simulink model "DLCReferenceApplication"  (R2023a)
settings: Solver=ode23tb  StartTime=0.0  StopTime=25  FixedStep=.001  RelTol=2e-1  EnableMultiTasking=on
StartFcn:
  | %tic
StopFcn:
  | %toc
model workspace (MAT data in the model file):
  DLCXref = [0 6.1 6.2 18 33 33.5 45 50 60]
  DLCXrefStanley = [0 1.2 2.4 3.6 4.8 6 7.2 8.4 9.44987166868 10.0991210544 10.1 10.1008789456 10.7501283313 11.8 15.24 18.68 22.12 25.56 29 31.0586706708 32.3317697631 32.5 33.2655829029 35.0745965915 36 38.7142857143 41.4285714286 44.1428571429 46.8571428571 49.5714285714 52.2857142857 55 55.7142857143 56.4285714286 57.1428571429 57.8571428571 58.5714285714 59.2857142857]
  DLCYref = [0 0 -5 -3.875 -3.5 1 0 0 0]
  DLCYrefStanley = [0.1375 0.1375 0.1375 0.1375 0.1375 0.1375 0.1375 0.1375 -0.203439148031 -1.09615705337 -2.2 -3.30384294663 -4.19656085197 -4.5375 -4.5375 -4.5375 -4.5375 -4.5375 -4.5375 -3.86895979121 -2.11844853934 -1.2 0.824587306188 2.01309074174 2.1375 1.85178571429 1.56607142857 1.28035714286 0.994642857143 0.708928571429 0.423214285714 0.1375 0.1375 0.1375 0.1375 0.1375 0.1375 0.1375]
  Downshift_Speeds = [9.5625  23.0625  36.5625  47.8125  59.0625  68.90625  78.75; 12.9375  26.4375  39.9375  51.1875  62.4375  72.84375  83.25; 16.3125  29.8125  43.3125  54.5625  65.8125  76.78125  87.75; 19.6875  33.1875  46.6875  57.9375  69.1875  80.71875  92.25]
  EngRevLim = 7000
  Pedal_Positions = [0.1 0.4 0.5 0.9]
  Upshift_Speeds = [12.9375  26.4375  39.9375  51.1875  62.4375  72.84375  83.25; 16.3125  29.8125  43.3125  54.5625  65.8125  76.78125  87.75; 19.6875  33.1875  46.6875  57.9375  69.1875  80.71875  92.25; 33  52.5  77.25  100.5  138.75  161.875  185]
  VEH.Mass = 1181
  VEH.StaticNormalFrontLoad.FR = 264.666666667
  VEH.StaticNormalFrontLoad.FL = 264.666666667
  VEH.StaticNormalRearLoad.RR = 322
  VEH.StaticNormalRearLoad.RL = 322
  VEH.WheelBase = 3.075
  VEH.FrontAxlePositionfromCG = 1.515
  VEH.RearAxlePositionfromCG = 1.504
  VEH.HeightCG = 0.134
  VEH.FrontalArea = 2.11
  VEH.DragCoefficient = 0.33
  VEH.NumberOfWheelsPerAxle = 2
  VEH.PitchMomentInertia = 1922.66666667
  VEH.RollMomentInertia = 432.333333333
  VEH.YawMomentInertia = 2066
  VEH.SteeringRatio = 18
  VEH.TrackWidth = 1.922
  VEH.SprungMass = 1096.72266667
  VEH.InitialLongPosition = 0
  VEH.InitialLatPosition = 5.7
  VEH.InitialVertPosition = 0
  VEH.InitialRollAngle = 0
  VEH.InitialPitchAngle = 0
  VEH.InitialYawAngle = 0
  VEH.InitialLongVel = 0
  VEH.InitialLatVel = 0
  VEH.InitialVertVel = 0
  VEH.InitialRollRate = 0
  VEH.InitialPitchRate = 0
  VEH.InitialYawRate = 0
  VEH.UnsprungMassRearAxle = 160
  VEH.UnsprungMassFrontAxle = 100
  rayDirections = [0  0  -1; 0  0  -1; 0  0  -1; 0  0  -1; 0  0  -1; 0  0  -1; 0  0  -1; 0  0  -1; 0  0  -1; 0  0  -1; 0  0  -1; 0  0  -1; 0  0  -1; 0  0  -1; 0  0  -1; 0  0  -1; 0  0  -1; 0  0  -1; 0  0  -1; 0  0  -1; 0  0  -1; 0  0  -1; 0  0  -1; 0  0  -1; 0  0  -1; 0  0  -1; 0  0  -1; 0  0  -1; 0  0  -1; 0  0  -1; 0  0  -1; 0  0  -1; 0  0  -1; 0  0  -1; 0  0  -1; 0  0  -1; 0  0  -1; 0  0  -1; 0  0  -1; 0  0  -1; 0  0  -1; 0  0  -1; 0  0  -1; 0  0  -1; 0  0  -1; 0  0  -1; 0  0  -1; 0  0  -1; 0  0  -1; 0  0  -1; 0  0  -1; 0  0  -1; 0  0  -1; 0  0  -1; 0  0  -1; 0  0  -1; 0  0  -1; 0  0  -1; 0  0  -1; 0  0  -1; 0  0  -1; 0  0  -1; 0  0  -1; 0  0  -1; 0  0  -1; 0  0  -1; 0  0  -1; 0  0  -1; 0  0  -1; 0  0  -1; 0  0  -1; 0  0  -1; 0  0  -1; 0  0  -1; 0  0  -1; 0  0  -1; 0  0  -1; 0  0  -1; 0  0  -1; 0  0  -1; 0  0  -1; 0  0  -1; 0  0  -1; 0  0  -1; 0  0  -1; 0  0  -1; 0  0  -1; 0  0  -1; 0  0  -1; 0  0  -1; 0  0  -1; 0  0  -1; 0  0  -1; 0  0  -1; 0  0  -1; 0  0  -1; 0  0  -1; 0  0  -1; 0  0  -1; 0  0  -1; 0  0  -1; 0  0  -1; 0  0  -1; 0  0  -1; 0  0  -1; 0  0  -1; 0  0  -1; 0  0  -1; 0  0  -1; 0  0  -1; 0  0  -1; 0  0  -1; 0  0  -1; 0  0  -1; 0  0  -1; 0  0  -1; 0  0  -1; 0  0  -1; 0  0  -1; 0  0  -1; 0  0  -1]
  rayLengths = [20; 20; 20; 20; 20; 20; 20; 20; 20; 20; 20; 20; 20; 20; 20; 20; 20; 20; 20; 20; 20; 20; 20; 20; 20; 20; 20; 20; 20; 20; 20; 20; 20; 20; 20; 20; 20; 20; 20; 20; 20; 20; 20; 20; 20; 20; 20; 20; 20; 20; 20; 20; 20; 20; 20; 20; 20; 20; 20; 20; 20; 20; 20; 20; 20; 20; 20; 20; 20; 20; 20; 20; 20; 20; 20; 20; 20; 20; 20; 20; 20; 20; 20; 20; 20; 20; 20; 20; 20; 20; 20; 20; 20; 20; 20; 20; 20; 20; 20; 20; 20; 20; 20; 20; 20; 20; 20; 20; 20; 20; 20; 20; 20; 20; 20; 20; 20; 20; 20; 20; 20]
  rayOrigins = [0.5  -0.5  0; 0.4  -0.5  0; 0.3  -0.5  0; 0.2  -0.5  0; 0.1  -0.5  0; 0  -0.5  0; -0.1  -0.5  0; -0.2  -0.5  0; -0.3  -0.5  0; -0.4  -0.5  0; -0.5  -0.5  0; 0.5  -0.4  0; 0.4  -0.4  0; 0.3  -0.4  0; 0.2  -0.4  0; 0.1  -0.4  0; 0  -0.4  0; -0.1  -0.4  0; -0.2  -0.4  0; -0.3  -0.4  0; -0.4  -0.4  0; -0.5  -0.4  0; 0.5  -0.3  0; 0.4  -0.3  0; 0.3  -0.3  0; 0.2  -0.3  0; 0.1  -0.3  0; 0  -0.3  0; -0.1  -0.3  0; -0.2  -0.3  0; -0.3  -0.3  0; -0.4  -0.3  0; -0.5  -0.3  0; 0.5  -0.2  0; 0.4  -0.2  0; 0.3  -0.2  0; 0.2  -0.2  0; 0.1  -0.2  0; 0  -0.2  0; -0.1  -0.2  0; -0.2  -0.2  0; -0.3  -0.2  0; -0.4  -0.2  0; -0.5  -0.2  0; 0.5  -0.1  0; 0.4  -0.1  0; 0.3  -0.1  0; 0.2  -0.1  0; 0.1  -0.1  0; 0  -0.1  0; -0.1  -0.1  0; -0.2  -0.1  0; -0.3  -0.1  0; -0.4  -0.1  0; -0.5  -0.1  0; 0.5  0  0; 0.4  0  0; 0.3  0  0; 0.2  0  0; 0.1  0  0; 0  0  0; -0.1  0  0; -0.2  0  0; -0.3  0  0; -0.4  0  0; -0.5  0  0; 0.5  0.1  0; 0.4  0.1  0; 0.3  0.1  0; 0.2  0.1  0; 0.1  0.1  0; 0  0.1  0; -0.1  0.1  0; -0.2  0.1  0; -0.3  0.1  0; -0.4  0.1  0; -0.5  0.1  0; 0.5  0.2  0; 0.4  0.2  0; 0.3  0.2  0; 0.2  0.2  0; 0.1  0.2  0; 0  0.2  0; -0.1  0.2  0; -0.2  0.2  0; -0.3  0.2  0; -0.4  0.2  0; -0.5  0.2  0; 0.5  0.3  0; 0.4  0.3  0; 0.3  0.3  0; 0.2  0.3  0; 0.1  0.3  0; 0  0.3  0; -0.1  0.3  0; -0.2  0.3  0; -0.3  0.3  0; -0.4  0.3  0; -0.5  0.3  0; 0.5  0.4  0; 0.4  0.4  0; 0.3  0.4  0; 0.2  0.4  0; 0.1  0.4  0; 0  0.4  0; -0.1  0.4  0; -0.2  0.4  0; -0.3  0.4  0; -0.4  0.4  0; -0.5  0.4  0; 0.5  0.5  0; 0.4  0.5  0; 0.3  0.5  0; 0.2  0.5  0; 0.1  0.5  0; 0  0.5  0; -0.1  0.5  0; -0.2  0.5  0; -0.3  0.5  0; -0.4  0.5  0; -0.5  0.5  0]
undefined symbols (not defined in the file or in its folder): DiscIntNeverNeededParam
libraries: simulink x14, autolibutils x7, vehdynlibdriver x2, vehdynlibviscommon x2, sim3dgroundtruthsensorlib x2, slpidlib x1, autolibtranscontrolscommon x1, autolibshared x1, sharedtransform x1, vehdynlibscenariocommon x1, vehdynlibsens x1, sim3dlib x1
(part 1 of 3)
settings Model: DataDictionary=DLCReferenceApplication.sldd  ModifiedByFormat=The MathWorks, Inc.  SimulationMode=accelerator  PacingRate=0.001000  Creator=The MathWorks, Inc.  LastModifiedBy=The MathWorks, Inc.
settings SolverCC: SolverJacobianMethodControl=FullPerturbation  ZeroCrossAlgorithm=Adaptive  AlgebraicLoopSolver=TrustRegion  AutoInsertRateTranBlk=on  InsertRTBMode=Never (minimum delay)  DecoupledContinuousIntegration=on  MinimalZcImpactIntegration=on  MaxZcPerStep=1
settings DataIOCC: ReturnWorkspaceOutputs=off
settings OptimizationCC: ReuseModelBlockBuffer=off
settings DebuggingCC: SignalInfNanChecking=error  ArtificialAlgebraicLoopMsg=none  MaskedZcDiagnostic=none  IgnoredZcDiagnostic=none  UnconnectedInputMsg=warning  UnconnectedOutputMsg=warning  UnconnectedLineMsg=warning  ModelReferenceExtraNoncontSigs=none  PregeneratedLibrarySubsystemCodeDiagnostic=none  ArithmeticOperatorsInVariantConditions=warning
settings ModelReferenceCC: UpdateModelReferenceTargets=IfOutOfDate  EnableRefExpFcnMdlSchedulingChecks=on  ModelReferenceMinAlgLoopOccurrences=on  PropagateSignalLabelsOutOfModel=off
settings SFSimCC: SimUseLocalCustomCode=off
settings RTWCC: RTWUseLocalCustomCode=off  DLArmComputeVersion=19.05

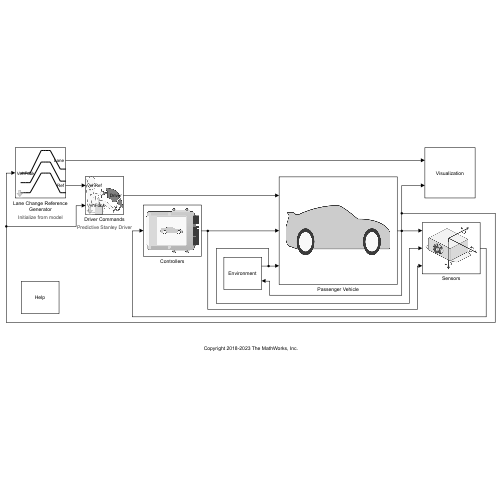
[thumbnail: Simulink's stored preview of the top-level diagram]
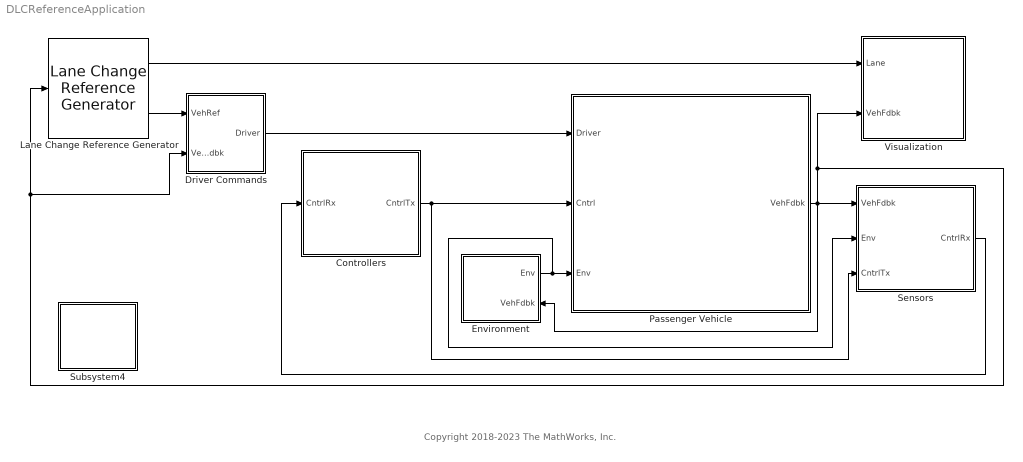
== system DLCReferenceApplication ==
  note: Copyright 2018-2023 The MathWorks, Inc.
  Controllers : Subsystem
      mask Display: image('SystemControllers.png')
  Driver Commands : Subsystem  VariantControl=0  mask(Driver Commands){driverType=Predictive Stanley Driver}
      mask prompts: driverType "Vehicle command mode"
      mask init:
      | [~]=vdynblksdrvrconfig(gcb)
      settings: AttributesFormatString=%<driverType>
      mask Help: eval('vdynblkshelp(''vdcrdriver'')');
      mask TypeOptions driverType: Longitudinal Driver | Predictive Driver | Predictive Stanley Driver | Open Loop
      mask Display: image('driverlatlong.png');
  Environment : Subsystem
      settings: PortSchema="{\"entries\":[{\"content\":{\"sides\":[{\"content\":{\"connectorIds\":[]},\"type\":\"ConnectorPlacement.EquallySpacedRectSide\",\"uuid\":\"7e477c5b-2979-4b31-83f8-8e06b5171f31\"},{\"content\":{\"connectorIds\":[\"Out1\",\"In1\"],\"side\":\"RIGHT\"},\"type\":\"ConnectorPlacement.EquallySpacedRectSide\",\"uuid\":\"d70ab29f-7073-466b-949c-fd6d019fdbd7\"},{\"content\":{\"connectorIds\":[],\"side\":\"TOP\"},\"type\":\"ConnectorPlacement.EquallySpacedRectSide\",\"uuid\":\"2d86cca8-a415-4272-bacd-17a50325dd7c\"}]},\"type\":\"ConnectorPlacement.EquallySpacedConnector\",\"uuid\":\"3f48fc9c-531e-41c0-b546-1206e5799aa8\"}],\"packageUris\":[\"http://schema.mathworks.com/mf0/Connector/R2020b\"],\"version\":\"1.0\"}"
      mask Display: disp('Environment')
  Lane Change Reference Generator : vehdynlibscenariocommon/Lane Change Reference Generator  ssMode=Initialize from model  ssVar=dlcSS35mph  t_start=1  XGate=175  xdot_r=35  xdotUnit=mph  xStart=2  vehW=2  latoff=VEH.InitialLatPosition  lattoff=VEH.InitialLatPosition  centerSwitch=on  xSimStop=off  ssDefault=on  latRefbp=DLCXrefStanley  latRef=DLCYrefStanley  X_o=175  Y_o=VEH.InitialLatPosition  psi_o=VEH.InitialYawAngle  ssTol=.15  ssMaxTime=30  ssWSName=dlcSS35mph  aMode=2  use3DCones=off
      settings: AttributesFormatString=%<ssMode>
  Passenger Vehicle : Subsystem
      mask Display: image('PassengerVehicle.png')
  Sensors : Subsystem
      mask Display: image('sensorimu.png'); % Use "Edit Image" on toolstrip to change.
  Subsystem4 : Subsystem
      settings: OpenFcn=eval('vdynblkshelp(''vdynblksdbllanechange'')');
      mask Display: disp('Help')
  Visualization : Subsystem
      mask Display: disp('Visualization')
  wires:
  Passenger Vehicle/1(VehFdbk) -> Lane Change Reference Generator/1, Driver Commands/2(VehFdbk), Visualization/2(VehFdbk), Environment/1(VehFdbk), Sensors/1(VehFdbk)
  Controllers/1(CntrlTx) -> Sensors/3(CntrlTx), Passenger Vehicle/2(Cntrl)
  Lane Change Reference Generator/1 -> Visualization/1(Lane)
  Driver Commands/1(Driver) -> Passenger Vehicle/1(Driver)
  Environment/1(Env) -> Passenger Vehicle/3(Env), Sensors/2(Env)
  Sensors/1(CntrlRx) -> Controllers/1(CntrlRx)
  Lane Change Reference Generator/2 -> Driver Commands/1(VehRef)

== system DLCReferenceApplication/Controllers ==
  CntrlRx : Inport
  Active Differential Control : Subsystem  Variant=on  VariantControlMode=label  LabelModeActiveChoice=0
  Brake Pressure Control : Subsystem  Variant=on  VariantControlMode=label  LabelModeActiveChoice=0
  Bus Creator : BusCreator  Inputs=1
  Bus Creator1 : BusCreator  Inputs=1
  Bus Creator2 : BusCreator  Inputs=3
  Bus Creator3 : BusCreator  Inputs=4
  Bus Creator4 : BusCreator  Inputs=1
  Bus Selector : BusSelector  OutputSignals=Driver.DecelFdbk,Wheels.Omega,IMU.Acc,Driver.AccFdbk,Wheels.BrkPrs
  Bus Selector1 : BusSelector  OutputSignals=Driver.AccFdbk,Driver.DecelFdbk,Driver.GearFdbk,Engine.EngSpd,Wheels.Omega
  Bus Selector2 : BusSelector  OutputSignals=Driver.AccFdbk,Engine.EngSpd
  Bus Selector3 : BusSelector  OutputSignals=Driver.AccFdbk,Driver.DecelFdbk,Driver.SteerFdbk,Driver.GearFdbk,Wheels.Omega,IMU.Acc,IMU.pqr
  ECU : Subsystem  SystemSampleTime=.01
  Ground : Ground
  Transmission Controller : Subsystem  Variant=on  VariantControlMode=label  VariantControl=Variant1  LabelModeActiveChoice=3
  CntrlTx : Outport  VectorParamsAs1DForOutWhenUnconnected=off
  wires:
  Bus Selector2/1 -> ECU/2(<Accel>)  "<AccFdbk>"
  Bus Creator/1 -> Bus Creator3/1  "ECU"
  Bus Creator1/1 -> Bus Creator3/2  "Transmission"
  Bus Creator3/1 -> CntrlTx/1  "CntrlTx"
  Bus Creator4/1 -> Bus Creator3/4  "Diff"
  Active Differential Control/1(DiffPrsCmd) -> Bus Creator4/1  "DiffPrsCmd"
  Active Differential Control/2(TrqCmd) -> [DiffTrqCmd]
  ECU/1(EngTrqCmd) -> Bus Creator/1  "EngTrqCmd"
  Transmission Controller/1(" Gear") -> Bus Creator1/1  "GearCmd"
  [DiffTrqCmd] -> ECU/1(DiffTrqCmd)  "DiffTrqCmd"
  Ground/1 -> Transmission Controller/7(UpReq), Transmission Controller/8(DownReq)
  Bus Selector2/2 -> ECU/3(EngSpd)  "<EngSpd>"
  Bus Selector1/5 -> Transmission Controller/5(Omega)  "<Omega>"
  Bus Selector1/2 -> Transmission Controller/2(BrkCmd)  "<DecelFdbk>"
  Bus Selector1/3 -> Transmission Controller/3(GearReq)  "<GearFdbk>"
  Bus Selector1/4 -> Transmission Controller/4(EngSpd)  "<EngSpd>"
  Bus Selector1/1 -> Transmission Controller/1(Accel)  "<AccFdbk>"
  Bus Selector3/1 -> Active Differential Control/1(Accel)  "<AccFdbk>"
  Bus Selector3/2 -> Active Differential Control/2(BrkCmd)  "<DecelFdbk>"
  Bus Selector3/3 -> Active Differential Control/3(Steer)  "<SteerFdbk>"
  Bus Selector3/4 -> Active Differential Control/4(GearFdbk)  "<GearFdbk>"
  Bus Selector3/5 -> Active Differential Control/5(Omega)  "<Omega>"
  Bus Selector3/6 -> Active Differential Control/6(axayaz)  "<Acc>"
  Bus Selector3/7 -> Active Differential Control/7(pqr)  "<pqr>"
  Bus Selector/1 -> Brake Pressure Control/1(DecelFdbk)  "<DecelFdbk>"
  CntrlRx/1 -> Bus Selector3/1, Bus Selector/1, Bus Selector1/1, Bus Selector2/1
  Bus Selector/2 -> Brake Pressure Control/2(Omega)  "<Omega>"
  Bus Selector/3 -> Brake Pressure Control/3(Accel)  "<Acc>"
  Brake Pressure Control/2(BrkPrsCmd) -> Bus Creator2/2  "BrkPrsCmd"
  Bus Creator2/1 -> Bus Creator3/3  "Brake"
  Brake Pressure Control/1(ABSFlag) -> [ABSFlag], Bus Creator2/1  "ABSFlag"
  [ABSFlag] -> Transmission Controller/6(ABSFlag)
  [ABSFlag] -> ECU/4(ABSFlag)
  Bus Selector/4 -> Brake Pressure Control/4(AccelFdbk)  "<AccFdbk>"
  Bus Selector/5 -> Brake Pressure Control/5(BrkPrs)  "<BrkPrs>"
  Brake Pressure Control/3(TCSFlag) -> Bus Creator2/3  "TCSFlag"

== system DLCReferenceApplication/Driver Commands ==
  VehRef : Inport
  VehFdbk : Inport  Port=2
  AccelGround : Ground
  BrakeGround : Ground
  Driver Commands : Subsystem  Variant=on  VariantControl=Variant1  AllowZeroVariantControls=on
  GearGround : Ground
  SteerGround : Ground
  Driver : Outport  VectorParamsAs1DForOutWhenUnconnected=off
  wires:
  VehRef/1 -> Driver Commands/1(VehRef)
  VehFdbk/1 -> Driver Commands/2(VehFdbk)
  Driver Commands/1(" Driver") -> Driver/1
  SteerGround/1 -> Driver Commands/3(SteerCmd)
  AccelGround/1 -> Driver Commands/4(Accel)
  BrakeGround/1 -> Driver Commands/5(Brake)
  GearGround/1 -> Driver Commands/6(Gear)

== system DLCReferenceApplication/Environment ==
  note: The Ground Feedback variant subsystem is automatically enabled/disabled according to the 3D Engine settings found in the Reference Generator.
      | Manually overriding this variant may result in initialization errors.
  VehFdbk : Inport
  Bus Creator1 : BusCreator  Inputs=2
  Constant3 : Constant  Value=0
  Constant4 : Constant  Value=0
  Constant5 : Constant  Value=0
  Friction : Constant  Value=ones(4,1).*1
  Ground Feedback : Subsystem  Variant=on  VariantControlMode=label  LabelModeActiveChoice=0
  Vector Concatenate : Concatenate  NumInputs=3
  Env : Outport  VectorParamsAs1DForOutWhenUnconnected=off
  wires:
  Constant5/1 -> Vector Concatenate/3  "Z"
  Vector Concatenate/1 -> Bus Creator1/1  "Wind"
  Constant3/1 -> Vector Concatenate/1  "X"
  Constant4/1 -> Vector Concatenate/2  "Y"
  Ground Feedback/1(Ground) -> Bus Creator1/2  "Gnd"
  Bus Creator1/1 -> Env/1
  Friction/1 -> Ground Feedback/1(Friction)
  VehFdbk/1 -> Ground Feedback/2(VehFdbk)

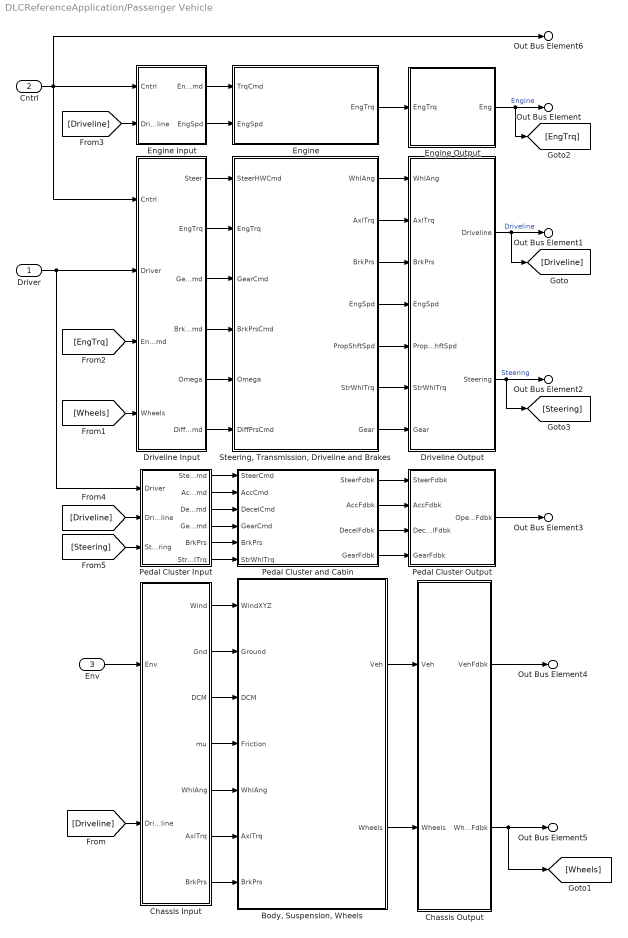
== system DLCReferenceApplication/Passenger Vehicle ==
  Driver : Inport
  Cntrl : Inport  Port=2
  Env : Inport  Port=3
  "Body, Suspension, Wheels" : Subsystem  Variant=on  VariantControlMode=label  LabelModeActiveChoice=3
  Chassis Input : Subsystem
  Chassis Output : Subsystem
  Driveline Input : Subsystem
  Driveline Output : Subsystem
  Engine : Subsystem  Variant=on  VariantControlMode=label  LabelModeActiveChoice=0
  Engine Input : Subsystem
  Engine Output : Subsystem
  Pedal Cluster Input : Subsystem
  Pedal Cluster Output : Subsystem
  Pedal Cluster and Cabin : Subsystem
  "Steering, Transmission, Driveline and Brakes" : Subsystem  Variant=on  VariantControlMode=label  LabelModeActiveChoice=0
  Out Bus Element : Outport  PortName=VehFdbk  Element=Engine
  Out Bus Element1 : Outport  PortName=VehFdbk  Element=Driveline
  Out Bus Element2 : Outport  PortName=VehFdbk  Element=Steering
  Out Bus Element3 : Outport  PortName=VehFdbk  Element=Driver
  Out Bus Element4 : Outport  PortName=VehFdbk  Element=Body
  Out Bus Element5 : Outport  PortName=VehFdbk  Element=Wheels
  Out Bus Element6 : Outport  PortName=VehFdbk  Element=Cntrl
  wires:
  Env/1 -> Chassis Input/1(Env)
  Chassis Input/1(Wind) -> "Body, Suspension, Wheels"/1(WindXYZ)
  Chassis Input/2(Gnd) -> "Body, Suspension, Wheels"/2(Ground)
  Chassis Input/4(mu) -> "Body, Suspension, Wheels"/4(Friction)
  Chassis Input/5(WhlAng) -> "Body, Suspension, Wheels"/5(WhlAng)
  Chassis Input/6(AxlTrq) -> "Body, Suspension, Wheels"/6(AxlTrq)
  Chassis Input/7(BrkPrs) -> "Body, Suspension, Wheels"/7(BrkPrs)
  Driveline Output/1(Driveline) -> Out Bus Element1/1, [Driveline]  "Driveline"
  "Steering, Transmission, Driveline and Brakes"/1(WhlAng) -> Driveline Output/1(WhlAng)
  "Steering, Transmission, Driveline and Brakes"/2(AxlTrq) -> Driveline Output/2(AxlTrq)
  "Steering, Transmission, Driveline and Brakes"/3(BrkPrs) -> Driveline Output/3(BrkPrs)
  "Steering, Transmission, Driveline and Brakes"/4(EngSpd) -> Driveline Output/4(EngSpd)
  "Steering, Transmission, Driveline and Brakes"/5(PropShftSpd) -> Driveline Output/5(PropShftSpd)
  Driver/1 -> Pedal Cluster Input/1(Driver), Driveline Input/2(Driver)
  Cntrl/1 -> Out Bus Element6/1, Engine Input/1(Cntrl), Driveline Input/1(Cntrl)
  Driveline Input/1(Steer) -> "Steering, Transmission, Driveline and Brakes"/1(SteerHWCmd)
  Driveline Input/3(GearCmd) -> "Steering, Transmission, Driveline and Brakes"/3(GearCmd)
  Driveline Input/4(BrkPrsCmd) -> "Steering, Transmission, Driveline and Brakes"/4(BrkPrsCmd)
  Driveline Input/5(Omega) -> "Steering, Transmission, Driveline and Brakes"/5(Omega)
  Engine/1(EngTrq) -> Engine Output/1("EngTrq ")
  Driveline Input/2(EngTrq) -> "Steering, Transmission, Driveline and Brakes"/2(EngTrq)
  Engine Input/1(EngTrqCmd) -> Engine/1(TrqCmd)
  Engine Input/2(EngSpd) -> Engine/2(EngSpd)
  Engine Output/1(Eng) -> Out Bus Element/1, [EngTrq]  "Engine"
  [Driveline] -> Chassis Input/2(Driveline)
  [Wheels] -> Driveline Input/4(Wheels)
  [EngTrq] -> Driveline Input/3(EngTrqCmd)
  [Driveline] -> Engine Input/2(Driveline)
  Driveline Input/6(DiffPrsCmd) -> "Steering, Transmission, Driveline and Brakes"/6(DiffPrsCmd)
  "Steering, Transmission, Driveline and Brakes"/6(StrWhlTrq) -> Driveline Output/6(StrWhlTrq)
  Driveline Output/2(Steering) -> Out Bus Element2/1, [Steering]  "Steering"
  Pedal Cluster Output/1(OperatorFdbk) -> Out Bus Element3/1
  Pedal Cluster and Cabin/1(SteerFdbk) -> Pedal Cluster Output/1(SteerFdbk)
  Pedal Cluster and Cabin/2(AccFdbk) -> Pedal Cluster Output/2(AccFdbk)
  Pedal Cluster and Cabin/3(DecelFdbk) -> Pedal Cluster Output/3(DecelFdbk)
  Pedal Cluster and Cabin/4(GearFdbk) -> Pedal Cluster Output/4(GearFdbk)
  Pedal Cluster Input/4(GearCmd) -> Pedal Cluster and Cabin/4(GearCmd)
  Pedal Cluster Input/3(DecelCmd) -> Pedal Cluster and Cabin/3(DecelCmd)
  Pedal Cluster Input/2(AccelCmd) -> Pedal Cluster and Cabin/2(AccCmd)
  Pedal Cluster Input/1(SteerCmd) -> Pedal Cluster and Cabin/1(SteerCmd)
  [Driveline] -> Pedal Cluster Input/2(Driveline)
  Pedal Cluster Input/5(BrkPrs) -> Pedal Cluster and Cabin/5(BrkPrs)
  [Steering] -> Pedal Cluster Input/3(Steering)
  Pedal Cluster Input/6(StrWhlTrq) -> Pedal Cluster and Cabin/6(StrWhlTrq)
  "Body, Suspension, Wheels"/2(Wheels) -> Chassis Output/2(Wheels)
  "Body, Suspension, Wheels"/1(Veh) -> Chassis Output/1(Veh)
  Chassis Output/2(WheelsFdbk) -> [Wheels], Out Bus Element5/1
  Chassis Output/1(VehFdbk) -> Out Bus Element4/1
  "Steering, Transmission, Driveline and Brakes"/7(Gear) -> Driveline Output/7(Gear)
  Chassis Input/3(DCM) -> "Body, Suspension, Wheels"/3(DCM)

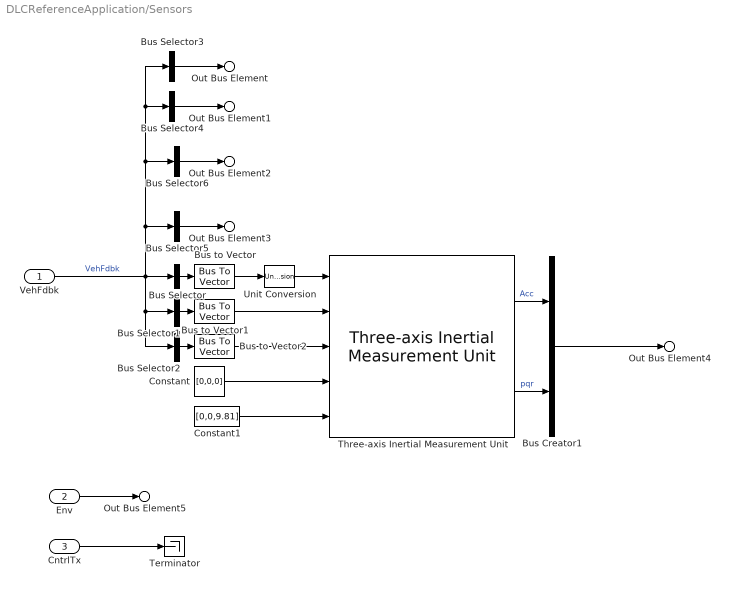
== system DLCReferenceApplication/Sensors ==
  VehFdbk : Inport
  Env : Inport  Port=2
  CntrlTx : Inport  Port=3
  Bus Creator1 : BusCreator  Inputs=2
  Bus Selector : BusSelector  OutputSignals=Body.BdyFrm.Cg.Acc.ax,Body.BdyFrm.Cg.Acc.ay,Body.BdyFrm.Cg.Acc.az  OutputAsBus=on
  Bus Selector1 : BusSelector  OutputSignals=Body.BdyFrm.Cg.AngVel.p,Body.BdyFrm.Cg.AngVel.q,Body.BdyFrm.Cg.AngVel.r  OutputAsBus=on
  Bus Selector2 : BusSelector  OutputSignals=Body.BdyFrm.Cg.AngAcc.pdot,Body.BdyFrm.Cg.AngAcc.qdot,Body.BdyFrm.Cg.AngAcc.rdot  OutputAsBus=on
  Bus Selector3 : BusSelector  OutputSignals=Driver  OutputAsBus=on
  Bus Selector4 : BusSelector  OutputSignals=Engine.EngTrq,Driveline.EngSpd  OutputAsBus=on
  Bus Selector5 : BusSelector  OutputSignals=Driveline.BrkPrs,Wheels.TireFrame.Kappa,Wheels.TireFrame.Alpha,Wheels.TireFrame.Omega  OutputAsBus=on
  Bus Selector6 : BusSelector  OutputSignals=Driveline.PropShftSpd,Driveline.AxlTrq  OutputAsBus=on
  Bus to Vector : BusToVector
  Bus to Vector1 : BusToVector
  Bus to Vector2 : BusToVector
  Constant : Constant  Value=[0,0,0]
  Constant1 : Constant  Value=[0,0,9.81]
  Terminator : Terminator
  Three-axis Inertial Measurement Unit : vehdynlibsens/Three-axis Inertial Measurement Unit  units=Metric (MKS)  imu=[0 0 0]  i_Ts=0  dtype_a=off  w_a=190  z_a=0.707  a_sf_cc=[1 0 0; 0 1 0; 0 0 1]  a_bias=[0 0 0]  a_sat="[-inf  -inf  -inf  inf inf inf]"  dtype_g=off  w_g=190  z_g=0.707  g_sf_cc=[1 0 0; 0 1 0; 0 0 1]  g_bias=[0 0 0]  g_sens=[0 0 0]  g_sat="[-inf  -inf  -inf  inf inf inf]"  i_rand=on  i_seeds=[23093 23094 23095 23096 23097 23098]  i_pow=[0.001 0.001 0.001 0.0001 0.0001 0.0001]  aMode=2
  Unit Conversion : UnitConversion
  Out Bus Element : Outport  PortName=CntrlRx  Element=Driver
  Out Bus Element1 : Outport  PortName=CntrlRx  Element=Engine
  Out Bus Element2 : Outport  PortName=CntrlRx  Element=Trans
  Out Bus Element3 : Outport  PortName=CntrlRx  Element=Wheels
  Out Bus Element4 : Outport  PortName=CntrlRx  Element=IMU
  Out Bus Element5 : Outport  PortName=CntrlRx  Element=Env
  wires:
  VehFdbk/1 -> Bus Selector/1, Bus Selector2/1, Bus Selector1/1, Bus Selector6/1, Bus Selector3/1, Bus Selector4/1, Bus Selector5/1  "VehFdbk"
  Bus Creator1/1 -> Out Bus Element4/1
  Three-axis Inertial Measurement Unit/1 -> Bus Creator1/1  "Acc"
  Three-axis Inertial Measurement Unit/2 -> Bus Creator1/2  "pqr"
  Bus Selector/1 -> Bus to Vector/1
  Bus to Vector/1 -> Unit Conversion/1
  Bus Selector1/1 -> Bus to Vector1/1
  Bus to Vector1/1 -> Three-axis Inertial Measurement Unit/2
  Env/1 -> Out Bus Element5/1
  Bus Selector2/1 -> Bus to Vector2/1
  Bus to Vector2/1 -> Three-axis Inertial Measurement Unit/3
  Constant/1 -> Three-axis Inertial Measurement Unit/4
  Constant1/1 -> Three-axis Inertial Measurement Unit/5
  Unit Conversion/1 -> Three-axis Inertial Measurement Unit/1
  CntrlTx/1 -> Terminator/1
  Bus Selector3/1 -> Out Bus Element/1
  Bus Selector4/1 -> Out Bus Element1/1
  Bus Selector5/1 -> Out Bus Element3/1
  Bus Selector6/1 -> Out Bus Element2/1

== system DLCReferenceApplication/Subsystem4 ==

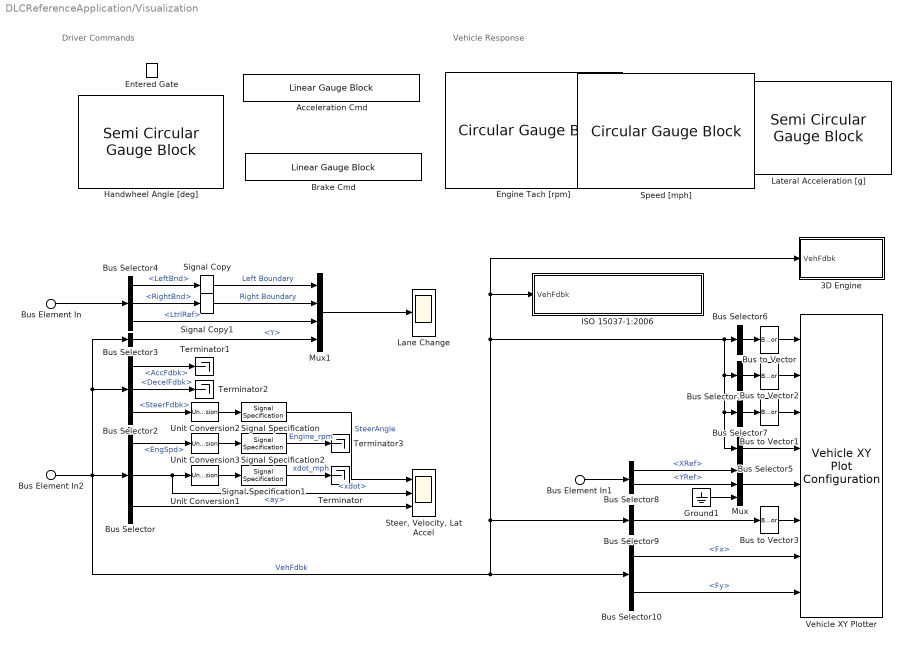
== system DLCReferenceApplication/Visualization ==
  note: Vehicle Response
  note: Driver Commands
  Bus Element In : Inport  PortName=Lane
  Bus Element In1 : Inport  PortName=Lane
  Bus Element In2 : Inport  Port=2  PortName=VehFdbk
  3D Engine : Subsystem  Variant=on  mask(3D Engine){engine3D=Disabled, use3DOp=off, SceneDesc=Double lane change, dt3D=.03, defaultPos=Recommended for scene, X_o=0, Y_o=5.7, Z_o=0, phi_o=0, theta_o=0, psi_o=0}
      mask prompts: engine3D "vdynblks:vehdynRefApp3DEng:blkPrm_engine3D"; use3DOp "Use default operating point"; SceneDesc "shared_sim3dblks:sim3dblkConfig:SceneDesc"; dt3D "vdynblks:vehdynRefApp3DEng:blkPrm_dt3D"; X_o "vdynblks:vehdynRefApp3DEng:blkPrm_X_o"; Y_o "vdynblks:vehdynRefApp3DEng:blkPrm_Y_o"; Z_o "vdynblks:vehdynRefApp3DEng:blkPrm_Z_o"; phi_o "vdynblks:vehdynRefApp3DEng:blkPrm_phi_o"; theta_o "vdynblks:vehdynRefApp3DEng:blkPrm_theta_o"; psi_o "vdynblks:vehdynRefApp3DEng:blkPrm_psi_o"
      mask help: This subsystem contains the interface blocks which permit the display of the vehicle in the 3D virtual environment. Enable it to view the simulation progress, disable it to inhibit the display.
      mask init:
      | GrndFdbkPath = find_system(bdroot(gcb), 'MatchFilter', @Simulink.match.allVariants,'BlockType','SubSystem','Name','Ground Feedback');
      | ManBlkName = 'Lane Change Reference Generator';
      | ManBlkPath = find_system(bdroot(gcb), 'MatchFilter', @Simulink.match.allVariants,'BlockType','SubSystem','Name',ManBlkName);
      | OpVarName = 'dlcSS35mph';
      | switch get_param(gcb,'engine3D')    
      |     case 'Disabled'
      |         try
      |             set_param(GrndFdbkPath{:},'OverrideUsingVariant','0');
      |         catch
      |             disp('Warning: Ground feedback source subsystem was not found. Ground feedback source remains unchanged.')
      |         end
      |         try
      |             if strcmp(get_param(gcb,'use3DOp'),'on') && strcmp(get_param(ManBlkPath{:},'ssMode'),'Resume from a workspace variable')
      |                 set_param(ManBlkPath{:},'ssVar',OpVarName);
      |             end
      |         catch
      |              disp('Warning: Maneuver source block not found. Steady state operating point not set')
      |         end
      |     case 'Enabled'
      |         try
      |             set_param(GrndFdbkPath{:},'OverrideUsingVariant','1');            
      |         catch
      |             disp('Warning: Ground feedback source subsystem was not found. Ground feedback source remains unchanged.')
      |         end
      |         try
      |             if strcmp(get_param(gcb,'use3DOp'),'on') && strcmp(get_param(ManBlkPath{:},'ssMode'),'Resume from a workspace variable')
      |                 set_param(ManBlkPath{:},'ssVar',[OpVarName '3D']);
      |             end
      |         catch
      |              disp('Warning: Maneuver source block not found. Steady state operating point not set')
      |         end
      |     otherwise
      | end
      settings: AttributesFormatString=|
      | %<SceneDesc>
      | %<engine3D>
      mask Help: eval('vdynblkshelp(''vdynblks3dengine'')');
      mask TypeOptions engine3D: vdynblks:vehdynRefApp3DEng:blkRdBt_engine3D_c1 | vdynblks:vehdynRefApp3DEng:blkRdBt_engine3D_c2
      mask Callback engine3D:
      | ManBlkName = 'Lane Change Reference Generator';
      | ManBlkPath = find_system(bdroot(gcb),'MatchFilter', @Simulink.match.allVariants,'BlockType','SubSystem','Name',ManBlkName);
      | switch get_param(gcb,'engine3D')
      |     case 'Disabled'
      |         try
      |             set_param(ManBlkPath{:},'use3DCones','off');
      |         catch
      |             disp('Warning: Lane change generator block not found in model')
      |         end
      |     case 'Enabled'
      |         try
      |             set_param(ManBlkPath{:},'use3DCones','on');
      |         catch
      |             disp('Warning: Lane change generator block not found in model')
      |         end
      |     otherwise
      | end
      mask TypeOptions SceneDesc: 3D Engine/Simulation 3D Scene Configuration/SceneDesc
      mask Callback SceneDesc:
      | defaultStatus = get_param(gcb,'defaultPos');
      | if strcmp(defaultStatus,'Recommended for scene')
      | sceneType = get_param(gcb,'SceneDesc');
      | switch sceneType
      |     case 'Straight road'
      |         set_param(gcb,'X_o', '-118')
      |         set_param(gcb,'Y_o', '5.7')
      |         set_param(gcb,'Z_o', '0')
      |         set_param(gcb,'phi_o', '0')
      |         set_param(gcb,'theta_o', '0')
      |         set_param(gcb,'psi_o', '0')
      |     case 'Curved road'
      |         set_param(gcb,'X_o', '0.2')
      |         set_param(gcb,'Y_o', '-1605.0')
      |         set_param(gcb,'Z_o', '0')
      |         set_param(gcb,'phi_o', '0')
      |         set_param(gcb,'theta_o', '0')
      |         set_param(gcb,'psi_o', '-156*pi/180')
      |     case 'Parking lot'
      |         set_param(gcb,'X_o', '-104.0')
      |         set_param(gcb,'Y_o', '-9.7')
      |         set_param(gcb,'Z_o', '0')
      |         set_param(gcb,'phi_o', '0')
      |         set_param(gcb,'theta_o', '0')
      |         set_param(gcb,'psi_o', '0')
      |     case 'Double lane change'
      |         set_param(gcb,'X_o', '0')
      |         set_param(gcb,'Y_o', '5.7')
      |         set_param(gcb,'Z_o', '0')
      |         set_param(gcb,'phi_o', '0')
      |         set_param(gcb,'theta_o', '0')
      |         set_param(gcb,'psi_o', '0')
      |     case 'Open surface'
      |         set_param(gcb,'X_o', '0')
      |         set_param(gcb,'Y_o', '0')
      |         set_param(gcb,'Z_o', '0')
      |         set_param(gcb,'phi_o', '0')
      |         set_param(gcb,'theta_o', '0')
      |         set_param(gcb,'psi_o', '0')
      |     case 'US highway'
      |         set_param(gcb,'X_o', '3592.00')
      |         set_param(gcb,'Y_o', '2617.00')
      |         set_param(gcb,'Z_o', '-1.0')
      |         set_param(gcb,'phi_o', '0')
      |         set_param(gcb,'theta_o', '0')
      |         set_param(gcb,'psi_o', '0')
      |     case 'US city block'
      |         set_param(gcb,'X_o', '-125.19')
      |         set_param(gcb,'Y_o', '1.65')
      |         set_param(gcb,'Z_o', '-0.04')
      |         set_param(gcb,'phi_o', '0')
      |         set_param(gcb,'theta_o', '0')
      |         set_param(gcb,'psi_o', '0')
      |     case 'Large parking lot'
      |         set_param(gcb,'X_o', '45.0')
      |         set_param(gcb,'Y_o', '54.7')
      |         set_param(gcb,'Z_o', '0.0')
      |         set_param(gcb,'phi_o', '0')
      |         set_param(gcb,'theta_o', '0')
      |         set_param(gcb,'psi_o', '-pi/2')
      |     case 'Virtual Mcity'
      |         set_param(gcb,'X_o', '-26.0')
      |         set_param(gcb,'Y_o', '76.0')
      |         set_param(gcb,'Z_o', '0.0')
      |         set_param(gcb,'phi_o', '0')
      |         set_param(gcb,'theta_o', '0')
      |         set_param(gcb,'psi_o', '-40*pi/180')
      |    case 'Suburban'
      |         set_param(gcb,'X_o', '60')
      |         set_param(gcb,'Y_o', '-41.7')
      |         set_param(gcb,'Z_o', '0.0')
      |         set_param(gcb,'phi_o', '0')
      |         set_param(gcb,'theta_o', '0')
      |         set_param(gcb,'psi_o', '-0.192')
      |     otherwise
      |         set_param(gcb,'X_o', '0')
      |         set_param(gcb,'Y_o', '0')
      |         set_param(gcb,'Z_o', '0')
      |         set_param(gcb,'phi_o', '0')
      |         set_param(gcb,'theta_o', '0')
      |         set_param(gcb,'psi_o', '0')
      | end
      | end
      mask TypeOptions defaultPos: vdynblks:vehdynRefApp3DEng:blkRdBt_defaultPos_c1 | vdynblks:vehdynRefApp3DEng:blkRdBt_defaultPos_c2
      mask DialogControl engineConfig Prompt: vdynblks:vehdynRefApp3DEng:blkDlg_engineConfig
      mask DialogControl engine3D Prompt: 3D Engine
      mask DialogControl SceneDesc Prompt: Scene name:
      mask DialogControl dt3D Prompt: 3D Engine frame rate, dt3D [s]:
      mask DialogControl posSetup Prompt: vdynblks:vehdynRefApp3DEng:blkDlg_posSetup
      mask DialogControl posSetupDesc Prompt: vdynblks:vehdynRefApp3DEng:blkDisTxt_posSetupDesc
      mask DialogControl X_o Prompt: Initial longitudinal position, X_o [m]:
      mask DialogControl Y_o Prompt: Initial lateral position, Y_o [m]:
      mask DialogControl Z_o Prompt: Initial vertical position, Z_o [m]:
      mask DialogControl phi_o Prompt: Initial roll angle, phi_o [rad]:
      mask DialogControl theta_o Prompt: Initial pitch angle, theta_o [rad]:
      mask DialogControl psi_o Prompt: Initial yaw angle, psi_o [rad]:
      mask DialogControl setModelPos Prompt: vdynblks:vehdynRefApp3DEng:blkDlg_setModelPos
      mask DialogControl setModelPos Callback:
      | if strcmp(get_param(bdroot(gcb),'SimulationStatus'),'stopped')
      |     sceneType = get_param(gcb,'SceneDesc');
      |     rootModel = bdroot(gcb);
      |     ws = get_param(rootModel, 'modelworkspace');
      |     VEH = getVariable(ws,'VEH');
      |     ParamList={'X_o',[1,1],{};'Y_o',[1,1],{};'Z_o',[1,1],{};'phi_o',[1,1],{'gte',-pi/2;'lte',pi/2};'theta_o',[1,1],{'gte',-pi/2;'lte',pi/2};'psi_o',[1,1],{'gte',-2*pi;'lte',2*pi}};
      |     paramStruct = autoblkscheckparams(gcb, '3D Engine',ParamList);
      |     VEH.InitialLongPosition = paramStruct.X_o;
      |     VEH.InitialLatPosition = paramStruct.Y_o;
      |     VEH.InitialVertPosition = paramStruct.Z_o;
      |     VEH.InitialRollAngle = paramStruct.phi_o;
      |     VEH.InitialPitchAngle = paramStruct.theta_o;
      |     VEH.InitialYawAngle = paramStruct.psi_o;
      |     assignin(ws,'VEH',VEH);
      |     modelList = {'PassVeh14DOF','PassVeh7DOF'};
      |     for idx =1:length(modelList)
      | %         try
      |             load_system(modelList{idx});
      |             ws = get_param(modelList{idx}, 'modelworkspace');
      |             assignin(ws,'VEH',VEH);
      |             save_system(modelList{idx});
      |             close_system(modelList{idx});
      | %         catch
      | %             disp(['Cannot find ' modelList{idx}])
      | %         end
      |     end
      | end
      mask Display: disp('3D Engine')
  Acceleration Cmd : LinearGaugeBlock  LabelPosition=Hide  ScaleMax=1  TickInterval=0.20000000000000001
  Brake Cmd : LinearGaugeBlock  LabelPosition=Hide  ScaleMax=1  TickInterval=0.20000000000000001
  Bus Selector : BusSelector  OutputSignals=Driveline.EngSpd,Body.BdyFrm.Cg.Vel.xdot,Body.BdyFrm.Cg.Acc.ay
  Bus Selector1 : BusSelector  OutputSignals=Body.InertFrm.Cg.Ang.phi,Body.InertFrm.Cg.Ang.theta,Body.InertFrm.Cg.Ang.psi  OutputAsBus=on
  Bus Selector10 : BusSelector  OutputSignals=Wheels.TireFrame.Fx,Wheels.TireFrame.Fy
  Bus Selector2 : BusSelector  OutputSignals=Driver.AccFdbk,Driver.DecelFdbk,Driver.SteerFdbk
  Bus Selector3 : BusSelector  OutputSignals=Body.InertFrm.Cg.Disp.Y
  Bus Selector4 : BusSelector  OutputSignals=LeftBnd,RightBnd,LtrlRef
  Bus Selector5 : BusSelector  OutputSignals=Driveline.WhlAng  OutputAsBus=on
  Bus Selector6 : BusSelector  OutputSignals=Body.InertFrm.Geom.Disp.X,Body.InertFrm.Geom.Disp.Y,Body.InertFrm.Geom.Disp.Z  OutputAsBus=on
  Bus Selector7 : BusSelector  OutputSignals=Body.InertFrm.Geom.Vel.Xdot,Body.InertFrm.Geom.Vel.Ydot,Body.InertFrm.Geom.Vel.Zdot  OutputAsBus=on
  Bus Selector8 : BusSelector  OutputSignals=XRef,YRef
  Bus Selector9 : BusSelector  OutputSignals=Driveline.EngSpd,Driveline.Gear  OutputAsBus=on
  Bus to Vector{,1..3} (4 alike) : BusToVector
  Engine Tach [rpm] : CircularGaugeBlock  LabelPosition=Hide  ScaleMax=8000  TickInterval=1000
  Entered Gate : LampBlock  LabelPosition=Hide
  Ground1 : Ground
  Handwheel Angle [deg] : SemiCircularGaugeBlock  LabelPosition=Hide  ScaleMin=-300  ScaleMax=300  TickInterval=60
  ISO 15037-1:2006 : Subsystem  StopFcn=|  Variant=on  VariantControlMode=label  LabelModeActiveChoice=0  mask(ISO 15037-1:2006){Measurement=Disabled}
      | switch get_param(gcb,'Measurement')
      |     case 'Enabled'
      |        p=slproject.getCurrentProject;
      |        projectRoot=p.RootFolder;
      |        SySFolder=fullfile(projectRoot, 'System');
      |        Simulink.sdi.loadView([SySFolder filesep 'ISO15037_1_2006E.mldatx']);
      |        Simulink.sdi.view;
      | end
      mask prompts: Measurement "ISO Measurements"
      mask help: Enables display of ISO 15037-1:2006 standard measurement signals in the Simulation Data Inspector.
      mask init:
      | switch get_param(gcb,'Measurement')
      |     case 'Disabled'
      |         set_param(gcb,'OverrideUsingVariant','0')
      |     case 'Enabled'
      |        set_param(gcb,'OverrideUsingVariant','1')
      |     otherwise
      |        set_param(gcb,'OverrideUsingVariant','0')
      | end
      settings: AttributesFormatString=%<Measurement>
      mask Help: eval('vdynblkshelp(''iso15037'')');
      mask TypeOptions Measurement: Enabled | Disabled
      mask Callback Measurement:
      | switch get_param(gcb,'Measurement')
      |     case 'Disabled'
      |         set_param(gcb,'OverrideUsingVariant','0')
      |     case 'Enabled'
      |        set_param(gcb,'OverrideUsingVariant','1')
      |     otherwise
      |        set_param(gcb,'OverrideUsingVariant','0')
      | end
      mask Display: disp('ISO 15037-1:2006')
  Lane Change : Scope
  Lateral Acceleration [g] : SemiCircularGaugeBlock  LabelPosition=Hide  ScaleMin=-1  ScaleMax=1  TickInterval=0.5
  Mux : Mux  Inputs=3
  Mux1 : Mux
  Signal Copy : SignalConversion  OverrideOpt=off
  Signal Copy1 : SignalConversion  OverrideOpt=off
  Signal Specification : SignalSpecification  Unit=deg
  Signal Specification1 : SignalSpecification  Unit=mph
  Signal Specification2 : SignalSpecification  Unit=rpm
  Speed [mph] : CircularGaugeBlock  LabelPosition=Hide  TickInterval=10
  "Steer, Velocity, Lat Accel" : Scope  NumInputPorts=3
  Terminator{,1..3} (4 alike) : Terminator
  Unit Conversion1 : UnitConversion
  Unit Conversion2 : UnitConversion
  Unit Conversion3 : UnitConversion
  Vehicle XY Plotter : vehdynlibviscommon/Vehicle XY Plot Configuration  extRef=on  extStats=on  extTireF=on  a=VEH.FrontAxlePositionfromCG  b=VEH.RearAxlePositionfromCG  w=VEH.TrackWidth  figBorder=10  bufferSize=1024  velNorm=5  tireFNorm=1000  pltDT=.1
  wires:
  Signal Specification/1 -> "Steer, Velocity, Lat Accel"/1  "SteerAngle"
  Bus Selector/3 -> "Steer, Velocity, Lat Accel"/3  "<ay>"
  Bus Selector/2 -> "Steer, Velocity, Lat Accel"/2, Unit Conversion1/1  "<xdot>"
  Unit Conversion2/1 -> Signal Specification/1
  Unit Conversion1/1 -> Signal Specification1/1
  Signal Specification1/1 -> Terminator/1  "xdot_mph"
  Bus Selector4/2 -> Signal Copy1/1  "<RightBnd>"
  Mux1/1 -> Lane Change/1
  Bus Selector3/1 -> Mux1/4  "<Y>"
  Bus Selector4/1 -> Signal Copy/1  "<LeftBnd>"
  Bus Selector4/3 -> Mux1/3  "<LtrlRef>"
  Bus Selector2/3 -> Unit Conversion2/1  "<SteerFdbk>"
  Bus Selector2/1 -> Terminator1/1  "<AccFdbk>"
  Bus Selector2/2 -> Terminator2/1  "<DecelFdbk>"
  Signal Specification2/1 -> Terminator3/1  "Engine_rpm"
  Unit Conversion3/1 -> Signal Specification2/1
  Bus Selector/1 -> Unit Conversion3/1  "<EngSpd>"
  Bus Selector7/1 -> Bus to Vector1/1
  Bus to Vector/1 -> Vehicle XY Plotter/1
  Bus Selector6/1 -> Bus to Vector/1
  Bus to Vector1/1 -> Vehicle XY Plotter/3
  Bus Selector1/1 -> Bus to Vector2/1
  Bus Element In2/1 -> Bus Selector3/1, Bus Selector2/1, ISO 15037-1:2006/1(VehFdbk), 3D Engine/1(VehFdbk), Bus Selector5/1, Bus Selector7/1, Bus Selector1/1, Bus Selector6/1, Bus Selector9/1, Bus Selector10/1, Bus Selector/1  "VehFdbk"
  Mux/1 -> Vehicle XY Plotter/5
  Ground1/1 -> Mux/3
  Bus Selector8/1 -> Mux/1  "<XRef>"
  Bus Element In/1 -> Bus Selector4/1
  Bus Selector8/2 -> Mux/2  "<YRef>"
  Bus to Vector3/1 -> Vehicle XY Plotter/6
  Bus Selector9/1 -> Bus to Vector3/1
  Bus to Vector2/1 -> Vehicle XY Plotter/2
  Bus Selector5/1 -> Vehicle XY Plotter/4
  Bus Selector10/2 -> Vehicle XY Plotter/8  "<Fy>"
  Bus Selector10/1 -> Vehicle XY Plotter/7  "<Fx>"
  Signal Copy/1 -> Mux1/1  "Left Boundary"
  Signal Copy1/1 -> Mux1/2  "Right Boundary"
  Bus Element In1/1 -> Bus Selector8/1

== system DLCReferenceApplication/Controllers/Active Differential Control ==
  note: 1) Add Subsystem or Model blocks as valid variant choices.
      | 2) You cannot connect blocks at this level. At simulation, connectivity is automatically
      | determined, based on the active variant and port name matching.
  Accel : Inport
  BrkCmd : Inport  Port=2
  Steer : Inport  Port=3
  GearFdbk : Inport  Port=4
  Omega : Inport  Port=5  Unit=rad/s
  axayaz : Inport  Port=6
  pqr : Inport  Port=7
  No Control : Subsystem  VariantControl=0
  Rear Diff Controller : Subsystem  TreatAsAtomicUnit=on  SystemSampleTime=.01  VariantControl=1
  DiffPrsCmd : Outport  VectorParamsAs1DForOutWhenUnconnected=off
  TrqCmd : Outport  Port=2  VectorParamsAs1DForOutWhenUnconnected=off

== system DLCReferenceApplication/Controllers/Brake Pressure Control ==
  note: 1) Add Subsystem or Model blocks as valid variant choices.
      | 2) You cannot connect blocks at this level. At simulation, connectivity is automatically
      | determined, based on the active variant and port name matching.
  DecelFdbk : Inport
  Omega : Inport  Port=2
  Accel : Inport  Port=3
  AccelFdbk : Inport  Port=4
  BrkPrs : Inport  Port=5
  Bang Bang ABS : Subsystem  VariantControl=1
  Five-State ABS and TCS : Subsystem  VariantControl=2
  Open Loop : Subsystem  VariantControl=0
  ABSFlag : Outport  VectorParamsAs1DForOutWhenUnconnected=off
  BrkPrsCmd : Outport  Port=2  VectorParamsAs1DForOutWhenUnconnected=off
  TCSFlag : Outport  Port=3  VectorParamsAs1DForOutWhenUnconnected=off

== system DLCReferenceApplication/Controllers/ECU ==
  DiffTrqCmd : Inport
  <Accel> : Inport  Port=2
  EngSpd : Inport  Port=3
  ABSFlag : Inport  Port=4
  First Order Hold : FirstOrderHold  ErrorTolerance=100
  Torque Cmd : Subsystem  TreatAsAtomicUnit=on  SystemSampleTime=.01
  EngTrqCmd : Outport  VectorParamsAs1DForOutWhenUnconnected=off
  wires:
  First Order Hold/1 -> EngTrqCmd/1
  DiffTrqCmd/1 -> Torque Cmd/1(DiffTrqCmd)
  <Accel>/1 -> Torque Cmd/2(<Accel>)
  EngSpd/1 -> Torque Cmd/3(EngSpd)
  Torque Cmd/1(EngTrqCmd) -> First Order Hold/1
  ABSFlag/1 -> Torque Cmd/4(ABSFlag)

== system DLCReferenceApplication/Controllers/Transmission Controller ==
  Accel : Inport
  BrkCmd : Inport  Port=2
  GearReq : Inport  Port=3
  EngSpd : Inport  Port=4
  Omega : Inport  Port=5  Unit=rad/s
  ABSFlag : Inport  Port=6
  UpReq : Inport  Port=7
  DownReq : Inport  Port=8  Unit=rad/s
  Driver - No Clutch : Subsystem  VariantControl=1
  PRNDL Controller : Subsystem  VariantControl=3
  Paddles : Subsystem  VariantControl=2
  Transmission Controller : Subsystem  VariantControl=0
  " Gear" : Outport  VectorParamsAs1DForOutWhenUnconnected=off

== system DLCReferenceApplication/Driver Commands/Driver Commands ==
  VehRef : Inport
  VehFdbk : Inport  Port=2
  SteerCmd : Inport  Port=3
  Accel : Inport  Port=4
  Brake : Inport  Port=5
  Gear : Inport  Port=6
  Longitudinal Driver : Subsystem  VariantControl=driverType==1
  Open Loop : Subsystem  VariantControl=driverType==4
  Predictive Driver : Subsystem  VariantControl=driverType==2
  Predictive Stanley Driver : Subsystem  VariantControl=driverType==3
  " Driver" : Outport  VectorParamsAs1DForOutWhenUnconnected=off

== system DLCReferenceApplication/Environment/Ground Feedback ==
  Friction : Inport
  VehFdbk : Inport  Port=2
  3D Engine : Subsystem  VariantControl=1
  Constant : Subsystem  VariantControl=0
  Ground : Outport  VectorParamsAs1DForOutWhenUnconnected=off

== system DLCReferenceApplication/Passenger Vehicle/Body, Suspension, Wheels ==
  note: 1) Add additional chassis Model reference blocks as valid variant choices for your specific use cases.
      | 2) You cannot connect blocks at this level. At simulation, connectivity is automatically
      | determined, based on the active variant and port name matching.
  WindXYZ : Inport
  Ground : Inport  Port=2  PortDimensions=4
  DCM : Inport  Port=3
  Friction : Inport  Port=4  PortDimensions=4
  WhlAng : Inport  Port=5
  AxlTrq : Inport  Port=6
  BrkPrs : Inport  Port=7
  PassVeh14DOF : ModelReference  DisableCoverage=on  ModelNameDialog=PassVeh14DOF  VariantControl=3  ModelReferenceVersion=6.11
  PassVeh7DOF : ModelReference  ModelNameDialog=PassVeh7DOF  SimulationMode=Normal  VariantControl=1  ModelReferenceVersion=6.2
  Veh : Outport  VectorParamsAs1DForOutWhenUnconnected=off
  Wheels : Outport  Port=2  VectorParamsAs1DForOutWhenUnconnected=off

== system DLCReferenceApplication/Passenger Vehicle/Chassis Input ==
  Env : Inport
  Driveline : Inport  Port=2
  Bus Selector1 : BusSelector  OutputSignals=Gnd.z.G_FL_z,Gnd.z.G_FR_z,Gnd.z.G_RL_z,Gnd.z.G_RR_z
  Bus Selector2 : BusSelector  OutputSignals=Wind
  Bus Selector3 : BusSelector  OutputSignals=Gnd.mu.mu_FL,Gnd.mu.mu_FR,Gnd.mu.mu_RL,Gnd.mu.mu_RR
  Bus Selector4 : BusSelector  OutputSignals=WhlAng,AxlTrq,BrkPrs
  Bus Selector5 : BusSelector  OutputSignals=Gnd.DCM
  Vector Concatenate : Concatenate  NumInputs=4
  Vector Concatenate1 : Concatenate  NumInputs=4
  Wind : Outport  VectorParamsAs1DForOutWhenUnconnected=off
  Gnd : Outport  Port=2  VectorParamsAs1DForOutWhenUnconnected=off
  DCM : Outport  Port=3  VectorParamsAs1DForOutWhenUnconnected=off
  mu : Outport  Port=4  VectorParamsAs1DForOutWhenUnconnected=off
  WhlAng : Outport  Port=5  VectorParamsAs1DForOutWhenUnconnected=off
  AxlTrq : Outport  Port=6  VectorParamsAs1DForOutWhenUnconnected=off
  BrkPrs : Outport  Port=7  VectorParamsAs1DForOutWhenUnconnected=off
  wires:
  Env/1 -> Bus Selector5/1, Bus Selector3/1, Bus Selector1/1, Bus Selector2/1
  Bus Selector2/1 -> Wind/1  "<Wind>"
  Bus Selector3/1 -> Vector Concatenate/1  "<mu_FL>"
  Bus Selector3/2 -> Vector Concatenate/2  "<mu_FR>"
  Bus Selector3/3 -> Vector Concatenate/3  "<mu_RL>"
  Bus Selector3/4 -> Vector Concatenate/4  "<mu_RR>"
  Vector Concatenate/1 -> mu/1
  Bus Selector1/1 -> Vector Concatenate1/1  "<G_FL_z>"
  Bus Selector1/2 -> Vector Concatenate1/2  "<G_FR_z>"
  Bus Selector1/3 -> Vector Concatenate1/3  "<G_RL_z>"
  Bus Selector1/4 -> Vector Concatenate1/4  "<G_RR_z>"
  Vector Concatenate1/1 -> Gnd/1
  Driveline/1 -> Bus Selector4/1
  Bus Selector4/2 -> AxlTrq/1  "<AxlTrq>"
  Bus Selector4/1 -> WhlAng/1  "<WhlAng>"
  Bus Selector4/3 -> BrkPrs/1  "<BrkPrs>"
  Bus Selector5/1 -> DCM/1  "<DCM>"

== system DLCReferenceApplication/Passenger Vehicle/Chassis Output ==
  Veh : Inport
  Wheels : Inport  Port=2
  Out Bus Element4 : Outport  PortName=VehFdbk
  Out Bus Element1 : Outport  Port=2  PortName=WheelsFdbk
  wires:
  Veh/1 -> Out Bus Element4/1
  Wheels/1 -> Out Bus Element1/1

== system DLCReferenceApplication/Passenger Vehicle/Driveline Input ==
  Cntrl : Inport
  Driver : Inport  Port=2
  EngTrqCmd : Inport  Port=3
  Wheels : Inport  Port=4
  Bus Selector1 : BusSelector  OutputSignals=SteerCmd
  Bus Selector2 : BusSelector  OutputSignals=TireFrame.Omega
  Bus Selector3 : BusSelector  OutputSignals=Transmission.GearCmd,Brake.BrkPrsCmd,Diff.DiffPrsCmd
  Bus Selector4 : BusSelector  OutputSignals=EngTrq
  Data Type Conversion : DataTypeConversion  SaturateOnIntegerOverflow=off  RndMeth=Floor
  Steer : Outport  VectorParamsAs1DForOutWhenUnconnected=off
  EngTrq : Outport  Port=2  VectorParamsAs1DForOutWhenUnconnected=off
  GearCmd : Outport  Port=3  VectorParamsAs1DForOutWhenUnconnected=off
  BrkPrsCmd : Outport  Port=4  VectorParamsAs1DForOutWhenUnconnected=off
  Omega : Outport  Port=5  VectorParamsAs1DForOutWhenUnconnected=off
  DiffPrsCmd : Outport  Port=6  VectorParamsAs1DForOutWhenUnconnected=off
  wires:
  Cntrl/1 -> Bus Selector3/1
  Bus Selector3/1 -> Data Type Conversion/1  "<GearCmd>"
  Driver/1 -> Bus Selector1/1
  Wheels/1 -> Bus Selector2/1
  Bus Selector2/1 -> Omega/1  "<Omega>"
  Bus Selector3/2 -> BrkPrsCmd/1  "<BrkPrsCmd>"
  EngTrqCmd/1 -> Bus Selector4/1
  Bus Selector1/1 -> Steer/1  "<SteerCmd>"
  Bus Selector4/1 -> EngTrq/1  "<EngTrq>"
  Bus Selector3/3 -> DiffPrsCmd/1  "<DiffPrsCmd>"
  Data Type Conversion/1 -> GearCmd/1

== system DLCReferenceApplication/Passenger Vehicle/Driveline Output ==
  WhlAng : Inport
  AxlTrq : Inport  Port=2
  BrkPrs : Inport  Port=3
  EngSpd : Inport  Port=4
  PropShftSpd : Inport  Port=5
  StrWhlTrq : Inport  Port=6
  Gear : Inport  Port=7
  Bus Creator1 : BusCreator  Inputs=6
  Bus Creator2 : BusCreator  Inputs=1
  Driveline : Outport  VectorParamsAs1DForOutWhenUnconnected=off
  Steering : Outport  Port=2  VectorParamsAs1DForOutWhenUnconnected=off
  wires:
  Bus Creator1/1 -> Driveline/1  "Driveline"
  PropShftSpd/1 -> Bus Creator1/5  "PropShftSpd"
  AxlTrq/1 -> Bus Creator1/2  "AxlTrq"
  WhlAng/1 -> Bus Creator1/1  "WhlAng"
  EngSpd/1 -> Bus Creator1/4  "EngSpd"
  BrkPrs/1 -> Bus Creator1/3  "BrkPrs"
  StrWhlTrq/1 -> Bus Creator2/1  "StrWhlTrq"
  Bus Creator2/1 -> Steering/1  "Steering"
  Gear/1 -> Bus Creator1/6  "Gear"

== system DLCReferenceApplication/Passenger Vehicle/Engine ==
  note: 1) Add additional Engine Model reference blocks as valid variant choices for your specific use cases.
      | 2) You cannot connect blocks at this level. At simulation, connectivity is automatically
      | determined, based on the active variant and port name matching.
  TrqCmd : Inport
  EngSpd : Inport  Port=2  Unit=rad/s
  Ideal Mapped Engine : ModelReference  DisableCoverage=on  ModelNameDialog=SiMappedEngineV  VariantControl=0  ModelReferenceVersion=6.0
  EngTrq : Outport  VectorParamsAs1DForOutWhenUnconnected=off

== system DLCReferenceApplication/Passenger Vehicle/Engine Input ==
  Cntrl : Inport
  Driveline : Inport  Port=2
  Bus Selector : BusSelector  OutputSignals=ECU.EngTrqCmd
  Bus Selector1 : BusSelector  OutputSignals=EngSpd
  EngTrqCmd : Outport  VectorParamsAs1DForOutWhenUnconnected=off
  EngSpd : Outport  Port=2  VectorParamsAs1DForOutWhenUnconnected=off
  wires:
  Driveline/1 -> Bus Selector1/1
  Cntrl/1 -> Bus Selector/1
  Bus Selector/1 -> EngTrqCmd/1  "<EngTrqCmd>"
  Bus Selector1/1 -> EngSpd/1  "<EngSpd>"

== system DLCReferenceApplication/Passenger Vehicle/Engine Output ==
  "EngTrq " : Inport
  Bus Creator : BusCreator  Inputs=1
  Eng : Outport  VectorParamsAs1DForOutWhenUnconnected=off
  wires:
  "EngTrq "/1 -> Bus Creator/1  "EngTrq"
  Bus Creator/1 -> Eng/1
